simulink library "vmc"  (R2021b)
settings: Solver=VariableStepAuto  StartTime=0.0  StopTime=10.0  RelTol=1e-3
undefined symbols (not defined in the file or in its folder): AVMC_ACCDeltaTqIGain_X_kph, AVMC_ACCDeltaTqIGain_Y_mps2, AVMC_ACCDeltaTqPGain_X_kph, AVMC_ACCDeltaTqPGain_Y_kph, AVMC_ACCLongSteadyCtrl_X_kph, AVMC_AggressJerkPCT4AT_X_kph, AVMC_AggressJerkPCT_X_kph, AVMC_AggressLimitPCT4AT_X_kph, AVMC_AggressLimitPCT_X_kph, AVMC_CCLongSteadyCtrl_X_kph, AVMC_DISCDeltaTqIGain_X_kph, AVMC_DISCDeltaTqIGain_Y_mps2, AVMC_DISCDeltaTqPGain_X_kph, AVMC_DISCDeltaTqPGain_Y_kph, AVMC_DISCTrunAccJerk_X_s, AVMC_DISCTrunAccLimit_X_s, AVMC_ESCRegenOut_X_kph, AVMC_ESCRegenOut_Y_Deg, AVMC_ESCRegenOutEnSpd_X_Deg, AVMC_ISOAccLimit_X_mps, AVMC_ISODecLimit_X_mps, AVMC_ISOJerk_X_mps, AVMC_LatESCRegenOut_X_kph, AVMC_LatESCRegenOut_Y_Deg, AVMC_LongAccDeadZone_X_kph, AVMC_LongAccFiltTsforP2_X_Gps, AVMC_MCPresBaseTq_X_bar, AVMC_MSALongSteadyCtrl_X_kph, AVMC_MSAPedalOvrd2_X_kph, AVMC_MSAPedalOvrd_X_kph, AVMC_MSASpdBand_X_kph, AVMC_MSATqDownEndTq_X_kph, AVMC_MSATqDownTime_X_kph, AVMC_RDCDetectTime_X_kph, AVMC_RDCDetectTime_Y_pct, AVMC_RDCEnSlideRate_X_Deg, AVMC_RearWhlTqRatio_X_Nm, AVMC_RearWhlTqRatio_Y_gps, AVMC_RearWhlTqSlipGain_X_rat, AVMC_RearWhlTqSlipGain_Y_kph, AVMC_SoftJerkPCT_X_kph, AVMC_SoftLimitPCT_X_kph, AVMC_StESCYaw_X_kph, AVMC_StESCYaw_Y_Deg, AVMC_StESCYawCom_X_kph, AVMC_StESCYawCom_Y_Gps, AVMC_TMSpdBaseTq_X_rpm, AVMC_VehHoldBDecMap_X_kph, AVMC_VehHoldDecCtrlTime_X_kph, AVMC_VehHoldMCPPass_X_deg, C_TASK_10MS_S, C_TASK_5MS_S, DEG2RAD, Discrete, ENUM_ACCAVAIL_AVAILABLE, ENUM_ACCCTRLALLOW_ALLOW, ENUM_ADASACCSTA_ACTIVE, ENUM_ADASACCSTA_OVERRIDE, ENUM_ADASACCSTA_SHUTOFF, ENUM_ADASAEBREQ_NOREQUEST ... (+361)
libraries: hcu_lib x63, simulink x60, simulink_extras x3, ctrlSharedLib x3, $bdroot x2
(part 1 of 15)
settings Model: Creator=FVT22120  LastModifiedBy=FVT22063

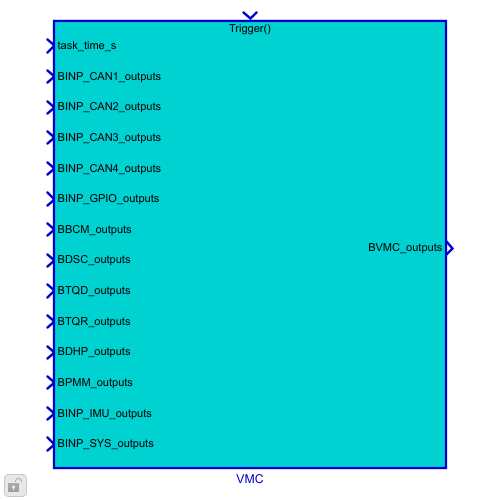
[thumbnail: Simulink's stored preview of the top-level diagram]
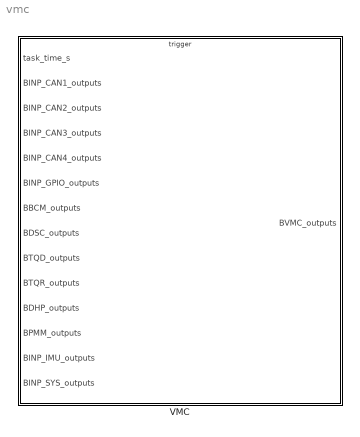
== system vmc ==
  VMC : Subsystem
      settings: RTWSystemCode=Nonreusable function  RTWFcnNameOpts=Use subsystem name  RTWFileNameOpts=Use subsystem name

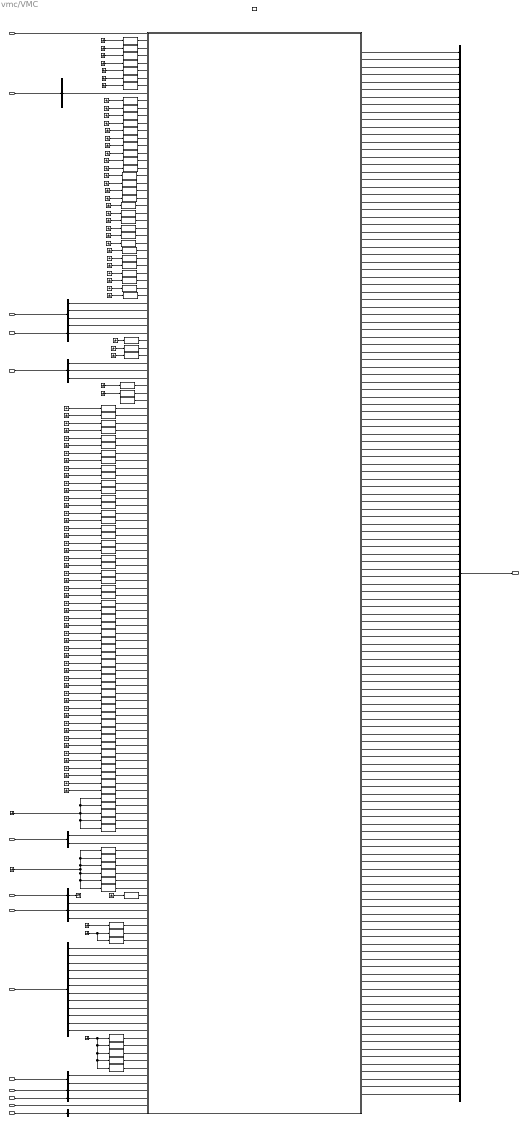
== system vmc/VMC ==
  task_time_s : Inport
  BINP_CAN1_outputs : Inport  Port=2  OutDataTypeStr=Bus: BINP_CAN1_outputs
  BINP_CAN2_outputs : Inport  Port=3  OutDataTypeStr=Bus: BINP_CAN2_outputs
  BINP_CAN3_outputs : Inport  Port=4  OutDataTypeStr=Bus: BINP_CAN3_outputs
  BINP_CAN4_outputs : Inport  Port=5  OutDataTypeStr=Bus: BINP_CAN4_outputs
  BINP_GPIO_outputs : Inport  Port=6  OutDataTypeStr=Bus: BINP_GPIO_outputs
  BBCM_outputs : Inport  Port=7  OutDataTypeStr=Bus: BBCM_outputs
  BDSC_outputs : Inport  Port=8  OutDataTypeStr=Bus: BDSC_outputs
  BTQD_outputs : Inport  Port=9  OutDataTypeStr=Bus: BTQD_outputs
  BTQR_outputs : Inport  Port=10  OutDataTypeStr=Bus: BTQR_outputs
  BDHP_outputs : Inport  Port=11  OutDataTypeStr=Bus: BDHP_outputs
  BPMM_outputs : Inport  Port=12  OutDataTypeStr=Bus: BPMM_outputs
  BINP_IMU_outputs : Inport  Port=13  OutDataTypeStr=Bus: BINP_IMU_outputs
  BINP_SYS_outputs : Inport  Port=14  OutDataTypeStr=Bus: BINP_SYS_outputs
  Trigger : TriggerPort  TriggerType=function-call  VariantControl=(inherit)  PortDimensions=1
  Bus Creator1 : BusCreator  Inputs=140  OutDataTypeStr=Bus: BVMC_outputs  NonVirtualBus=on
  Bus Selector1 : BusSelector  OutputSignals=VINP_SWCResUpSta_flg,VINP_SWCSetdownSta_flg,VINP_SWCCANCELSta_flg
  Bus Selector10 : BusSelector  OutputSignals=VDHP_ActAPSPosn_pct
  Bus Selector11 : BusSelector  OutputSignals=VPMM_DrivetrainSelect_enum
  Bus Selector12 : BusSelector  OutputSignals=VINP_DIDGetDynoMode_flg
  Bus Selector2 : BusSelector  OutputSignals=VBCM_HornCtrl_flg
  Bus Selector3 : BusSelector  OutputSignals=VDSC_DISCTurn_flg,VDSC_DISCSta_enum,VDSC_DISCTargetSpd_kph
  Bus Selector4 : BusSelector  OutputSignals=VTQD_DriverWhlTqDem_Nm,VTQD_CoordWhlTqDemFr_Nm,VTQD_CoordWhlTqDemRr_Nm,VTQD_GearActualPosn_enum,VTQD_ExternalTqAllow_flg,VTQD_LowIdleAccPedal_flg,VTQD_ExtShftAllow_flg,VTQD_FrEDUAvailBrkRgnTq_Nm,VTQD_RrEDUAvailBrkRgnTq_Nm,VTQD_AfterAvailableTqDemFr_Nm,VTQD_AfterAvailableTqDemRr_Nm,VTQD_ExtDoorAllow_flg
  Bus Selector5 : BusSelector  OutputSignals=VINP_RrTMSpd_rpm
  Bus Selector6 : BusSelector  OutputSignals=VINP_BrakeSWGPIO_flg,VINP_HoodSW_flg
  Bus Selector7 : BusSelector  OutputSignals=VINP_FASpeed_kph
  Bus Selector8 : BusSelector  OutputSignals=VINP_Distanceunit_flg,VINP_METERKPHCalcu_kph,VINP_GPSLAT_s,VINP_GPSLONG_enum
  Bus Selector9 : BusSelector  OutputSignals=VTQR_RrTMTqReq_Nm,VTQR_FrTMTqReq_Nm
  Cast To Boolean{,2..4,6..10,12..13,27,36} (13 alike) : DataTypeConversion  OutDataTypeStr=boolean
  Cast To Boolean{1,5,11,29..35} (10 alike) : DataTypeConversion  OutDataTypeStr=uint8
  Cast To Boolean{14..26,28,37} (15 alike) : DataTypeConversion  OutDataTypeStr=single
  Constant : Constant  Value=ZERO_INT
  Data Type Conversion{,1..24,55..57,62,64,68..69} (32 alike) : DataTypeConversion  OutDataTypeStr=uint8
  Data Type Conversion{25..42,44,53..54,60,63,67,70,72} (26 alike) : DataTypeConversion  OutDataTypeStr=boolean
  Data Type Conversion{43,45..52,61,65..66,71} (13 alike) : DataTypeConversion  OutDataTypeStr=single
  Data Type Conversion58 : DataTypeConversion  OutDataTypeStr=uint32
  Data Type Conversion59 : DataTypeConversion  OutDataTypeStr=uint32
  Ground{,1..96} (97 alike) : Ground
  Terminator : Terminator
  VMC : Subsystem
  BVMC_outputs : Outport  OutDataTypeStr=Bus:BVMC_outputs
  wires:
  BINP_CAN3_outputs/1 -> Bus Selector5/1
  Ground12/1 -> Data Type Conversion4/1
  Ground11/1 -> Data Type Conversion44/1
  Bus Selector4/7 -> VMC/129(VTQD_ExtShftAllow_flg)  "<VTQD_ExtShftAllow_flg>"
  Bus Selector4/6 -> VMC/128(VTQD_LowIdleAccPedal_flg)  "<VTQD_LowIdleAccPedal_flg>"
  Bus Selector8/1 -> VMC/37(VINP_Distanceunit_flg)  "<VINP_Distanceunit_flg>"
  Ground17/1 -> Data Type Conversion6/1
  Ground16/1 -> Data Type Conversion47/1
  Ground15/1 -> Data Type Conversion46/1
  Ground14/1 -> Data Type Conversion5/1
  Ground18/1 -> Data Type Conversion40/1
  Ground13/1 -> Data Type Conversion41/1
  Ground10/1 -> Data Type Conversion45/1
  Ground9/1 -> Data Type Conversion3/1
  Ground8/1 -> Data Type Conversion2/1
  Ground7/1 -> Data Type Conversion42/1
  Ground6/1 -> Data Type Conversion43/1
  Ground5/1 -> Data Type Conversion1/1
  Ground4/1 -> Data Type Conversion/1
  Bus Selector6/1 -> VMC/108(VINP_BrakeSWGPIO_flg)  "<VINP_BrakeSWGPIO_flg>"
  BINP_GPIO_outputs/1 -> Bus Selector6/1
  Ground3/1 -> Data Type Conversion65/1, Data Type Conversion64/1, Data Type Conversion63/1, Data Type Conversion60/1, Data Type Conversion61/1, Data Type Conversion62/1
  task_time_s/1 -> VMC/1(task_time_s)
  Bus Selector4/5 -> VMC/127(VTQD_ExternalTqAllow_flg)  "<VTQD_ExternalTqAllow_flg>"
  Bus Selector4/4 -> VMC/126(VTQD_GearActualPosn_enum)  "<VTQD_GearActualPosn_enum>"
  Bus Selector4/3 -> VMC/125(VTQD_CoordWhlTqDemRr_Nm)  "<VTQD_CoordWhlTqDemRr_Nm>"
  Bus Selector4/2 -> VMC/124(VTQD_CoordWhlTqDemFr_Nm)  "<VTQD_CoordWhlTqDemFr_Nm>"
  Bus Selector4/1 -> VMC/123(VTQD_DriverWhlTqDem_Nm)  "<VTQD_DriverWhlTqDem_Nm>"
  Bus Selector1/3 -> VMC/47(VINP_SWCCANCELSta_flg)  "<VINP_SWCCANCELSta_flg>"
  Bus Selector1/2 -> VMC/46(VINP_SWCSetdownSta_flg)  "<VINP_SWCSetdownSta_flg>"
  Bus Selector1/1 -> VMC/45(VINP_SWCResUpSta_flg)  "<VINP_SWCResUpSta_flg>"
  BTQD_outputs/1 -> Bus Selector4/1
  Bus Selector3/3 -> VMC/119(VDSC_DISCTargetSpd_kph)  "<VDSC_DISCTargetSpd_kph>"
  Bus Selector3/2 -> VMC/118(VDSC_DISCSta_enum)  "<VDSC_DISCSta_enum>"
  Bus Selector3/1 -> VMC/117(VDSC_DISCTurn_flg)  "<VDSC_DISCTurn_flg>"
  BDSC_outputs/1 -> Bus Selector3/1
  BBCM_outputs/1 -> Bus Selector2/1
  BINP_CAN4_outputs/1 -> Bus Selector1/1
  Bus Creator1/1 -> BVMC_outputs/1  "BVMC_outputs"
  BTQR_outputs/1 -> Bus Selector9/1
  Bus Selector9/1 -> VMC/140(VTQR_RrTMTqReq_Nm)  "<VTQR_RrTMTqReq_Nm>"
  Bus Selector4/9 -> VMC/131(VTQD_RrEDUAvailBrkRgnTq_Nm)  "<VTQD_RrEDUAvailBrkRgnTq_Nm>"
  Bus Selector4/10 -> VMC/132(VTQD_AfterAvailableTqDemFr_Nm)  "<VTQD_AfterAvailableTqDemFr_Nm>"
  Bus Selector4/11 -> VMC/133(VTQD_AfterAvailableTqDemRr_Nm)  "<VTQD_AfterAvailableTqDemRr_Nm>"
  BDHP_outputs/1 -> Bus Selector10/1
  Bus Selector10/1 -> VMC/142(VDHP_ActAPSPosn_pct)  "<VDHP_ActAPSPosn_pct>"
  VMC/1(VVMC_FeatSetSpdFinal_raw32) -> Bus Creator1/1
  VMC/2(VVMC_VehicleSpeed_mph) -> Bus Creator1/2
  VMC/3(VVMC_VehicleSpeed_kph) -> Bus Creator1/3
  VMC/4(VVMC_MeterIndSpeed_raw32) -> Bus Creator1/4
  VMC/5(VVMC_MeterIndSpeedForCalcu_kph) -> Bus Creator1/5
  VMC/6(VVMC_VMCAEBCtrlAvail_flg) -> Bus Creator1/6
  VMC/7(VVMC_VMCACCCtrlAvail_flg) -> Bus Creator1/7
  VMC/8(VVMC_VMCCCCtrlAvail_flg) -> Bus Creator1/8
  VMC/9(VVMC_VMCMSACtrlAvail_flg) -> Bus Creator1/9
  VMC/10(VVMC_FeatArbitrSta_enum) -> Bus Creator1/10
  VMC/11(VVMC_FeatReqSpd_kph) -> Bus Creator1/11
  VMC/12(VVMC_JerkPCT_pct) -> Bus Creator1/12
  VMC/13(VVMC_LimitPCT_pct) -> Bus Creator1/13
  VMC/14(VVMC_LFWhlSpeedRollAve_kph) -> Bus Creator1/14
  VMC/15(VVMC_RFWhlSpeedRollAve_kph) -> Bus Creator1/15
  VMC/16(VVMC_LRWhlSpeedRollAve_kph) -> Bus Creator1/16
  VMC/17(VVMC_RRWhlSpeedRollAve_kph) -> Bus Creator1/17
  VMC/18(VVMC_FrontRearSlipRatioCtrl_flg) -> Bus Creator1/18
  VMC/19(VVMC_RearWhlSlipRatioCtrl_flg) -> Bus Creator1/19
  VMC/20(VVMC_SingleWhlSlipRatioCtrl_flg) -> Bus Creator1/20
  VMC/21(VVMC_LatAccCtrl_flg) -> Bus Creator1/21
  VMC/22(VVMC_SafetyCtrl_flg) -> Bus Creator1/22
  VMC/23(VVMC_EstSlope_Deg) -> Bus Creator1/23
  VMC/24(VVMC_SPD2ACCAct_flg) -> Bus Creator1/24
  VMC/25(VVMC_AccCalcuPID_mps2) -> Bus Creator1/25
  VMC/26(VVMC_ISOAccLimit_mps2) -> Bus Creator1/26
  VMC/27(VVMC_ISODecLimit_mps2) -> Bus Creator1/27
  VMC/28(VVMC_ISOJerkLimit_mps3) -> Bus Creator1/28
  VMC/29(VVMC_ACCRequiredAccel_mps2) -> Bus Creator1/29
  VMC/30(VVMC_DISCReqAcc_mps2) -> Bus Creator1/30
  VMC/31(VVMC_FeatArbitrFinal_enum) -> Bus Creator1/31
  VMC/32(VVMC_ActACCRequiredAccel_mps2) -> Bus Creator1/32
  VMC/33(VVMC_LateralCtrl_flg) -> Bus Creator1/33
  VMC/34(VVMC_ADASLKASta_enum) -> Bus Creator1/34
  VMC/35(VVMC_LKAStrToqReq_Nm) -> Bus Creator1/35
  VMC/36(VVMC_LKATOIFault_flg) -> Bus Creator1/36
  VMC/37(VVMC_LKATOIAct_enum) -> Bus Creator1/37
  VMC/89(VVMC_ADASAEBSta_enum) -> Bus Creator1/89
  VMC/39(VVMC_ADASFaultSta_flg) -> Bus Creator1/39
  VMC/40(VVMC_AEBVehHoldReq_flg) -> Bus Creator1/40
  VMC/41(VVMC_ACCVehHoldReq_flg) -> Bus Creator1/41
  VMC/42(VVMC_ADASDBSReq_enum) -> Bus Creator1/42
  VMC/43(VVMC_ADASACCSta_enum) -> Bus Creator1/43
  VMC/44(VVMC_ACCObjDist_m) -> Bus Creator1/44
  VMC/45(VVMC_ACCObjRelSpd_mps) -> Bus Creator1/45
  VMC/46(VVMC_TimeGapLevel_enum) -> Bus Creator1/46
  VMC/47(VVMC_ACCJerkUpperLimit_mps3) -> Bus Creator1/47
  VMC/48(VVMC_ACCComfortBandUpper_mps2) -> Bus Creator1/48
  VMC/49(VVMC_ACCJerkLowerLimit_mps3) -> Bus Creator1/49
  VMC/50(VVMC_ACCComfortBandLower_mps2) -> Bus Creator1/50
  VMC/51(VVMC_ADASVehSpdLim_raw32) -> Bus Creator1/51
  VMC/52(VVMC_ADASShftPosnReqA_flg) -> Bus Creator1/52
  VMC/53(VVMC_ADASShftPosnReq_enum) -> Bus Creator1/53
  VMC/54(VVMC_ADASForceIdle_flg) -> Bus Creator1/54
  VMC/55(VVMC_HazardWarningReq_flg) -> Bus Creator1/55
  VMC/56(VVMC_RightTurnLightReq_flg) -> Bus Creator1/56
  VMC/57(VVMC_LeftTurnLightReq_flg) -> Bus Creator1/57
  VMC/58(VVMC_ADASFCWSta_enum) -> Bus Creator1/58
  VMC/59(VVMC_ADASLDWSta_enum) -> Bus Creator1/59
  VMC/60(VVMC_ADASFltWrnReq_flg) -> Bus Creator1/60
  VMC/61(VVMC_ACCObjDstLvl_enum) -> Bus Creator1/61
  VMC/62(VVMC_ForceLowBeam_enum) -> Bus Creator1/62
  VMC/63(VVMC_ACCTakeoverReq_flg) -> Bus Creator1/63
  VMC/64(VVMC_ADASWarningMsg_enum) -> Bus Creator1/64
  VMC/65(VVMC_ADASCAMSpdLim_enum) -> Bus Creator1/65
  VMC/66(VVMC_TargetType_enum) -> Bus Creator1/66
  VMC/67(VVMC_ADASSLIFSpdLim_enum) -> Bus Creator1/67
  VMC/68(VVMC_LKAHODDisplayWarning_flg) -> Bus Creator1/68
  VMC/69(VVMC_LKAHODSoundWarning_flg) -> Bus Creator1/69
  VMC/70(VVMC_ADASLFCSta_enum) -> Bus Creator1/70
  VMC/71(VVMC_ADASLaneModeL_enum) -> Bus Creator1/71
  VMC/72(VVMC_ADASLaneModeR_enum) -> Bus Creator1/72
  VMC/73(VVMC_ADASSLIFSta_enum) -> Bus Creator1/73
  VMC/74(VVMC_ADASISASta_enum) -> Bus Creator1/74
  VMC/75(VVMC_ADASLDWMute_flg) -> Bus Creator1/75
  VMC/76(VVMC_ADASFCWMute_flg) -> Bus Creator1/76
  VMC/77(VVMC_ADASLFCHandsOffWarning_enum) -> Bus Creator1/77
  VMC/78(VVMC_LVDADisabled_flg) -> Bus Creator1/78
  VMC/79(VVMC_LVDAMuteSta_enum) -> Bus Creator1/79
  VMC/80(VVMC_LVDAFailinfo_flg) -> Bus Creator1/80
  VMC/81(VVMC_LVDAWarning_flg) -> Bus Creator1/81
  VMC/82(VVMC_LVDAACCStatusInformation_flg) -> Bus Creator1/82
  VMC/83(VVMC_ADASLFCWarnSound_enum) -> Bus Creator1/83
  VMC/84(VVMC_FCMACCmode_enum) -> Bus Creator1/84
  VMC/85(VVMC_ADASLanetypeR_enum) -> Bus Creator1/85
  VMC/86(VVMC_ADASLanetypeL_enum) -> Bus Creator1/86
  VMC/87(VVMC_ADASLanecurveL_raw32) -> Bus Creator1/87
  VMC/88(VVMC_ADASLanecurveR_raw32) -> Bus Creator1/88
  VMC/38(VVMC_ADASAEBReq_enum) -> Bus Creator1/38
  VMC/90(VVMC_FCMLDWRequest_enum) -> Bus Creator1/90
  VMC/91(VVMC_FCMLDWFault_flg) -> Bus Creator1/91
  VMC/92(VVMC_ADASActive_flg) -> Bus Creator1/92
  VMC/93(VVMC_ACCCtrlAvail_flg) -> Bus Creator1/93
  VMC/94(VVMC_ADASNegReq_flg) -> Bus Creator1/94
  VMC/95(VVMC_ACCPedalOvrd_flg) -> Bus Creator1/95
  VMC/96(VVMC_ADASWhlTqReq_Nm) -> Bus Creator1/96
  VMC/97(VVMC_AccPedalOvrdDISC_flg) -> Bus Creator1/97
  VMC/98(VVMC_RearTqRatio_rat) -> Bus Creator1/98
  VMC/99(VVMC_TimeGapCalcu_s) -> Bus Creator1/99
  VMC/100(VVMC_CCCtrlSta_enum) -> Bus Creator1/100
  VMC/101(VVMC_CruzActive_flg) -> Bus Creator1/101
  VMC/102(VVMC_CCPedalOvrd_flg) -> Bus Creator1/102
  VMC/103(VVMC_CruzWhlTqReq_Nm) -> Bus Creator1/103
  VMC/104(VVMC_MSACtrlSta_enum) -> Bus Creator1/104
  VMC/105(VVMC_MSAActive_flg) -> Bus Creator1/105
  VMC/106(VVMC_MSAWhlTqReq_Nm) -> Bus Creator1/106
  VMC/107(VVMC_APSCtrlAvail_flg) -> Bus Creator1/107
  VMC/108(VVMC_APSActive_flg) -> Bus Creator1/108
  VMC/109(VVMC_APSSpeedCMD_kph) -> Bus Creator1/109
  VMC/110(VVMC_APSShiftPosnReq_enum) -> Bus Creator1/110
  VMC/111(VVMC_APSStaSys_enum) -> Bus Creator1/111
  VMC/112(VVMC_APSDecReqA_flg) -> Bus Creator1/112
  VMC/113(VVMC_APSDecReq_mps2) -> Bus Creator1/113
  VMC/114(VVMC_APSReq_enum) -> Bus Creator1/114
  VMC/115(VVMC_LongAcc_Gps) -> Bus Creator1/115
  VMC/116(VVMC_RawWhlSpdSlideRate_pct) -> Bus Creator1/116
  VMC/117(VVMC_LFWhlSpdSlideRate_pct) -> Bus Creator1/117
  VMC/118(VVMC_RFWhlSpdSlideRate_pct) -> Bus Creator1/118
  VMC/119(VVMC_LRWhlSpdSlideRate_pct) -> Bus Creator1/119
  VMC/120(VVMC_RRWhlSpdSlideRate_pct) -> Bus Creator1/120
  VMC/121(VVMC_PredictVehSpd_kph) -> Bus Creator1/121
  VMC/122(VVMC_LF4WhlSpdSlideRate_pct) -> Bus Creator1/122
  VMC/123(VVMC_RF4WhlSpdSlideRate_pct) -> Bus Creator1/123
  VMC/124(VVMC_LR4WhlSpdSlideRate_pct) -> Bus Creator1/124
  VMC/125(VVMC_RR4WhlSpdSlideRate_pct) -> Bus Creator1/125
  VMC/126(VVMC_4WhlSpdSlideRate_pct) -> Bus Creator1/126
  VMC/127(VVMC_ActMaxSlideRate_pct) -> Bus Creator1/127
  VMC/128(VVMC_ActLFSlideRate_pct) -> Bus Creator1/128
  VMC/129(VVMC_ActRFSlideRate_pct) -> Bus Creator1/129
  VMC/130(VVMC_ActLRSlideRate_pct) -> Bus Creator1/130
  VMC/131(VVMC_ActRRSlideRate_pct) -> Bus Creator1/131
  VMC/132(VVMC_AltLWhlSlideRate_pct) -> Bus Creator1/132
  VMC/133(VVMC_AltRWhlSlideRate_pct) -> Bus Creator1/133
  VMC/134(VVMC_AltWhlSlideRate_pct) -> Bus Creator1/134
  VMC/135(VVMC_CCMSASpdWar_flg) -> Bus Creator1/135
  Bus Selector9/2 -> VMC/141(VTQR_FrTMTqReq_Nm)  "<VTQR_FrTMTqReq_Nm>"
  Bus Selector4/8 -> VMC/130(VTQD_FrEDUAvailBrkRgnTq_Nm)  "<VTQD_FrEDUAvailBrkRgnTq_Nm>"
  Ground/1 -> Data Type Conversion59/1, Data Type Conversion58/1, Data Type Conversion55/1, Data Type Conversion56/1, Data Type Conversion57/1
  Bus Selector8/2 -> VMC/38(VINP_METERKPHCalcu_kph)  "<VINP_METERKPHCalcu_kph>"
  BINP_CAN2_outputs/1 -> Bus Selector8/1
  BPMM_outputs/1 -> Bus Selector11/1
  Bus Selector11/1 -> VMC/143(<VPMM_DrivetrainSelect_enum>)  "<VPMM_DrivetrainSelect_enum>"
  Constant/1 -> VMC/50(VINP_SCPSystemMode_enum)
  VMC/136(VVMC_IMUEnaCmd_flg) -> Bus Creator1/136
  VMC/137(VVMC_RWDRDCActive_enum) -> Bus Creator1/137
  Bus Selector4/12 -> VMC/134(VTQD_ExtDoorAllow_flg)  "<VTQD_ExtDoorAllow_flg>"
  VMC/138(VVMC_MSAWhlTqActive_flg) -> Bus Creator1/138
  Bus Selector5/1 -> VMC/41(VINP_RrTMSpd_rpm)  "<VINP_RrTMSpd_rpm>"
  BINP_IMU_outputs/1 -> VMC/144(BINP_IMU_outputs)
  VMC/139(VVMC_RDCEnSlideRate_pct) -> Bus Creator1/139
  VMC/140(VVMC_ActStESCYaw_Dps) -> Bus Creator1/140
  Bus Selector6/2 -> VMC/109(VINP_HoodSW_flg)  "<VINP_HoodSW_flg>"
  Bus Selector8/3 -> VMC/39(VINP_GPSLAT_sec)  "<VINP_GPSLAT_s>"
  Bus Selector8/4 -> VMC/40(VINP_GPSLONG_sec)  "<VINP_GPSLONG_enum>"
  BINP_SYS_outputs/1 -> Bus Selector12/1
  Bus Selector12/1 -> VMC/145(VINP_DIDGetDynoMode_flg)  "<VINP_DIDGetDynoMode_flg>"
  Ground1/1 -> Data Type Conversion66/1
  Ground2/1 -> Data Type Conversion53/1, Data Type Conversion54/1
  Data Type Conversion/1 -> VMC/51(VINP_ADASAEBSta_enum)
  Data Type Conversion1/1 -> VMC/52(VINP_ADASACCSta_enum)
  Data Type Conversion2/1 -> VMC/55(VINP_ADASAEBReq_enum)
  Data Type Conversion3/1 -> VMC/56(VINP_ADASLKASta_enum)
  Data Type Conversion4/1 -> VMC/59(VINP_LKATOIAct_enum)
  Data Type Conversion5/1 -> VMC/62(VINP_ADASDBSReq_enum)
  Data Type Conversion6/1 -> VMC/65(VINP_TimeGapLevel_enum)
  Data Type Conversion7/1 -> VMC/70(VINP_ForceLowBeam_enum)
  Data Type Conversion8/1 -> VMC/75(VINP_ADASVehSpdLim_raw32)
  Data Type Conversion9/1 -> VMC/77(VINP_ADASShftPosnReq_enum)
  Data Type Conversion10/1 -> VMC/78(VINP_ADASFCWSta_enum)
  Data Type Conversion11/1 -> VMC/79(VINP_ADASLDWSta_enum)
  Data Type Conversion12/1 -> VMC/81(VINP_ACCObjDstLvl_enum)
  Data Type Conversion13/1 -> VMC/83(VINP_ADASWarningMsg_enum)
  Data Type Conversion14/1 -> VMC/84(VINP_ADASCAMSpdLim_enum)
  Data Type Conversion15/1 -> VMC/85(VINP_TargetType_enum)
  Data Type Conversion16/1 -> VMC/86(VINP_ADASSLIFSpdLim_enum)
  Data Type Conversion17/1 -> VMC/89(VINP_ADASLFCSta_enum)
  Data Type Conversion18/1 -> VMC/90(VINP_ADASLaneModeL_enum)
  Data Type Conversion19/1 -> VMC/91(VINP_ADASLaneModeR_enum)
  Data Type Conversion20/1 -> VMC/92(VINP_ADASSLIFSta_enum)
  Data Type Conversion21/1 -> VMC/93(VINP_ADASISASta_enum)
  Data Type Conversion22/1 -> VMC/96(VINP_ADASLFCHandsOffWarning_enum)
  Data Type Conversion23/1 -> VMC/98(VINP_LVDAMuteSta_enum)
  Data Type Conversion24/1 -> VMC/102(VINP_ADASLFCWarnSound_enum)
  Data Type Conversion25/1 -> VMC/101(VINP_LVDAACCStatusInformation_flg)
  Data Type Conversion26/1 -> VMC/100(VINP_LVDAWarning_flg)
  Data Type Conversion27/1 -> VMC/99(VINP_LVDAFailinfo_flg)
  Data Type Conversion28/1 -> VMC/97(VINP_LVDADisabled_flg)
  Data Type Conversion29/1 -> VMC/95(VINP_ADASFCWMute_flg)
  Data Type Conversion30/1 -> VMC/94(VINP_ADASLDWMute_flg)
  Data Type Conversion31/1 -> VMC/88(VINP_LKAHODSoundWarning_flg)
  Data Type Conversion32/1 -> VMC/87(VINP_LKAHODDisplayWarning_flg)
  Data Type Conversion33/1 -> VMC/82(VINP_ACCTakeoverReq_flg)
  Data Type Conversion34/1 -> VMC/80(VINP_ADASFltWrnReq_flg)
  Data Type Conversion35/1 -> VMC/76(VINP_ADASShftPosnReqA_flg)
  Data Type Conversion36/1 -> VMC/69(VINP_LeftTurnLightReq_flg)
  Data Type Conversion37/1 -> VMC/68(VINP_RightTurnLightReq_flg)
  Data Type Conversion38/1 -> VMC/67(VINP_ADASForceIdle_flg)
  Data Type Conversion39/1 -> VMC/66(VINP_HazardWarningReq_flg)
  Data Type Conversion40/1 -> VMC/61(VINP_AEBVehHoldReq_flg)
  Data Type Conversion41/1 -> VMC/60(VINP_ADASFaultSta_flg)
  Data Type Conversion42/1 -> VMC/54(VINP_ACCVehHoldReq_flg)
  Data Type Conversion44/1 -> VMC/58(VINP_LKATOIFault_flg)
  Data Type Conversion43/1 -> VMC/53(VINP_ACCRequiredAccel_mps2)
  Data Type Conversion45/1 -> VMC/57(VINP_LKAStrToqReq_Nm)
  Data Type Conversion46/1 -> VMC/63(VINP_ACCObjDist_m)
  Data Type Conversion47/1 -> VMC/64(VINP_ACCObjRelSpd_mps)
  Data Type Conversion48/1 -> VMC/71(VINP_ACCJerkUpperLimit_mps3)
  Data Type Conversion49/1 -> VMC/72(VINP_ACCComfortBandUpper_mps2)
  Data Type Conversion50/1 -> VMC/73(VINP_ACCJerkLowerLimit_mps3)
  Data Type Conversion51/1 -> VMC/74(VINP_ACCComfortBandLower_mps2)
  Ground23/1 -> Data Type Conversion9/1
  Ground25/1 -> Data Type Conversion11/1
  Ground31/1 -> Data Type Conversion36/1
  Ground27/1 -> Data Type Conversion35/1
  Ground26/1 -> Data Type Conversion34/1
  Ground28/1 -> Data Type Conversion39/1
  Ground22/1 -> Data Type Conversion8/1
  Ground24/1 -> Data Type Conversion10/1
  Ground33/1 -> Data Type Conversion48/1
  Ground19/1 -> Data Type Conversion49/1
  Ground30/1 -> Data Type Conversion37/1
  Ground21/1 -> Data Type Conversion51/1
  Ground20/1 -> Data Type Conversion50/1
  Ground32/1 -> Data Type Conversion7/1
  Ground29/1 -> Data Type Conversion38/1
  Ground40/1 -> Data Type Conversion29/1
  Ground35/1 -> Data Type Conversion15/1
  Ground34/1 -> Data Type Conversion14/1
  Ground42/1 -> Data Type Conversion28/1
  Ground43/1 -> Data Type Conversion27/1
  Ground49/1 -> Data Type Conversion17/1
  Ground46/1 -> Data Type Conversion24/1
  Ground47/1 -> Data Type Conversion23/1
  Ground51/1 -> Data Type Conversion19/1
  Ground44/1 -> Data Type Conversion26/1
  Ground53/1 -> Data Type Conversion21/1
  Ground38/1 -> Data Type Conversion13/1
  Ground37/1 -> Data Type Conversion32/1
  Ground45/1 -> Data Type Conversion25/1
  Ground52/1 -> Data Type Conversion20/1
  Ground48/1 -> Data Type Conversion31/1
  Ground39/1 -> Data Type Conversion30/1
  Ground50/1 -> Data Type Conversion18/1
  Ground36/1 -> Data Type Conversion16/1
  Ground41/1 -> Data Type Conversion22/1
  Ground54/1 -> Data Type Conversion12/1
  Ground55/1 -> Data Type Conversion33/1
  Ground68/1 -> Cast To Boolean17/1
  Ground69/1 -> Cast To Boolean8/1
  Ground71/1 -> Cast To Boolean9/1
  Ground60/1 -> Cast To Boolean3/1
  Ground61/1 -> Cast To Boolean4/1
  Ground62/1 -> Cast To Boolean5/1
  Ground64/1 -> Cast To Boolean16/1
  Ground65/1 -> Cast To Boolean6/1
  Ground66/1 -> Cast To Boolean15/1
  Ground67/1 -> Cast To Boolean7/1
  Ground56/1 -> Cast To Boolean/1
  Ground57/1 -> Cast To Boolean14/1
  Ground58/1 -> Cast To Boolean2/1
  Ground59/1 -> Cast To Boolean1/1
  Ground75/1 -> Cast To Boolean21/1
  Ground81/1 -> Cast To Boolean24/1
  Ground82/1 -> Cast To Boolean25/1
  Ground72/1 -> Cast To Boolean19/1
  Ground83/1 -> Cast To Boolean26/1
  Ground74/1 -> Cast To Boolean20/1
  Ground87/1 -> Cast To Boolean30/1
  Ground76/1 -> Cast To Boolean22/1
  Ground78/1 -> Cast To Boolean12/1
  Ground86/1 -> Cast To Boolean29/1
  Ground79/1 -> Cast To Boolean13/1
  Ground84/1 -> Cast To Boolean27/1
  Ground73/1 -> Cast To Boolean10/1
  Ground77/1 -> Cast To Boolean11/1
  Ground85/1 -> Cast To Boolean28/1
  Ground80/1 -> Cast To Boolean23/1
  Ground88/1 -> Cast To Boolean31/1
  Ground89/1 -> Cast To Boolean32/1
  Ground90/1 -> Cast To Boolean33/1
  BINP_CAN1_outputs/1 -> Bus Selector7/1
  Ground91/1 -> Cast To Boolean37/1
  Ground93/1 -> Cast To Boolean35/1
  Ground92/1 -> Cast To Boolean36/1
  Ground94/1 -> Cast To Boolean34/1
  Ground95/1 -> Data Type Conversion52/1
  Bus Selector7/1 -> VMC/9(VINP_VehSpeed_kph)  "<VINP_FASpeed_kph>"
  Cast To Boolean/1 -> VMC/2(VINP_DriverSeatBeltCmd_flg)
  Cast To Boolean2/1 -> VMC/4(VINP_BrkSwSta_flg)
  Cast To Boolean1/1 -> VMC/5(VINP_EPBSta_enum)
  Cast To Boolean3/1 -> VMC/6(VINP_ACCAvail_flg)
  Cast To Boolean4/1 -> VMC/7(VINP_AEBAvail_flg)
  Cast To Boolean5/1 -> VMC/8(VINP_ESCOFFStatus_enum)
  Cast To Boolean6/1 -> VMC/11(VINP_LFRawWhlSpeedV_flg)
  Cast To Boolean7/1 -> VMC/13(VINP_RFRawWhlSpeedV_flg)
  Cast To Boolean8/1 -> VMC/15(VINP_LRRawWhlSpeedV_flg)
  Ground70/1 -> Cast To Boolean18/1
  Cast To Boolean9/1 -> VMC/17(VINP_RRRawWhlSpeedV_flg)
  Cast To Boolean10/1 -> VMC/19(VINP_LatAccelV_flg)
  Cast To Boolean11/1 -> VMC/23(VINP_ESCADASSta_enum)
  Cast To Boolean12/1 -> VMC/24(VINP_FrRBCActive_flg)
  Cast To Boolean13/1 -> VMC/25(VINP_RrRBCActive_flg)
  Cast To Boolean14/1 -> VMC/3(VINP_MeterIndVehSpeed_kph)
  Cast To Boolean16/1 -> VMC/10(VINP_LFRawWhlSpeed_kph)
  Cast To Boolean15/1 -> VMC/12(VINP_RFRawWhlSpeed_kph)
  Cast To Boolean17/1 -> VMC/14(VINP_LRRawWhlSpeed_kph)
  Cast To Boolean18/1 -> VMC/16(VINP_RRRawWhlSpeed_kph)
  Cast To Boolean19/1 -> VMC/18(VINP_LatAccel_Gps)
  Cast To Boolean20/1 -> VMC/20(VINP_GRADE_Deg)
  Cast To Boolean21/1 -> VMC/21(VINP_LongAccel_Gps)
  Cast To Boolean22/1 -> VMC/22(VINP_MCPressure_bar)
  Cast To Boolean23/1 -> VMC/26(VINP_FrntAxlTrqReqBrk_Nm)
  Cast To Boolean24/1 -> VMC/27(VINP_RearAxlTrqReqBrk_Nm)
  Cast To Boolean25/1 -> VMC/28(VINP_BrkPedalPos_pct)
  Cast To Boolean26/1 -> VMC/29(VINP_SASAngle_Deg)
  Cast To Boolean27/1 -> VMC/30(VINP_ESCActive_flg)
  Cast To Boolean28/1 -> VMC/31(VINP_YawRate_degps)
  Cast To Boolean29/1 -> VMC/32(VINP_RDCActive_enum)
  Cast To Boolean30/1 -> VMC/33(VINP_LFWhlRotDir_enum)
  Cast To Boolean31/1 -> VMC/34(VINP_LRWhlRotDir_enum)
  Cast To Boolean32/1 -> VMC/35(VINP_RFWhlRotDir_enum)
  Cast To Boolean33/1 -> VMC/36(VINP_RRWhlRotDir_enum)
  Data Type Conversion52/1 -> VMC/49(VINP_SetSpd_kph)
  Cast To Boolean34/1 -> VMC/48(VINP_RegenMode_enum)
  Cast To Boolean35/1 -> VMC/44(VINP_ZoneSpdCtrlMode_enum)
  Cast To Boolean36/1 -> VMC/43(VINP_ZoneSpdCtrlSta_flg)
  Cast To Boolean37/1 -> VMC/42(VINP_FrTMSpd_rpm)
  Data Type Conversion53/1 -> VMC/122(VDSC_AccDecResp_flg)
  Data Type Conversion54/1 -> VMC/121(VDSC_AutoTurnMode_flg)
  Data Type Conversion55/1 -> VMC/103(VINP_FCMACCmode_enum)
  Data Type Conversion56/1 -> VMC/104(VINP_ADASLanetypeR_enum)
  Data Type Conversion57/1 -> VMC/105(VINP_ADASLanetypeL_enum)
  Data Type Conversion58/1 -> VMC/106(VINP_ADASLanecurveL_raw32)
  Data Type Conversion59/1 -> VMC/107(VINP_ADASLanecurveR_raw32)
  Data Type Conversion60/1 -> VMC/110(APP_SpdLimit_flg)
  Data Type Conversion61/1 -> VMC/111(APP_SpdLimit)
  Data Type Conversion62/1 -> VMC/112(VAPS_APSStaSystem_enum)
  Data Type Conversion63/1 -> VMC/113(VAPS_APSVMCReqA_flg)
  Data Type Conversion64/1 -> VMC/114(VAPS_APSShiftPosnReq_enum)
  Data Type Conversion65/1 -> VMC/115(VAPS_APSSpeedCMD_kph)
  Data Type Conversion66/1 -> VMC/120(VDSC_TurningSpdMovingflat_kph)
  Data Type Conversion70/1 -> VMC/139(VTQD_EquivAccPedalSWSta_flg)
  Data Type Conversion69/1 -> VMC/138(VTQD_APSReq_enum)
  Data Type Conversion67/1 -> VMC/136(VTQD_APSDecReqA_flg)
  Data Type Conversion68/1 -> VMC/135(VTQD_APSStaSys_enum)
  Data Type Conversion71/1 -> VMC/137(VTQD_APSDecReq_mps2)
  Ground63/1 -> Data Type Conversion71/1, Data Type Conversion69/1, Data Type Conversion70/1, Data Type Conversion67/1, Data Type Conversion68/1
  Bus Selector2/1 -> Terminator/1  "<VBCM_HornCtrl_flg>"
  Data Type Conversion72/1 -> VMC/116(VBCM_DrDoorSW_flg)
  Ground96/1 -> Data Type Conversion72/1
